simulink model "SPWM"  (R2016b)
settings: Solver=VariableStepAuto  StartTime=0.0  StopTime=0.1  RelTol=1e-3
libraries: powerlib x7, powerlib_meascontrol x2
settings Model: Creator=sususweet  LastModifiedBy=tangyq

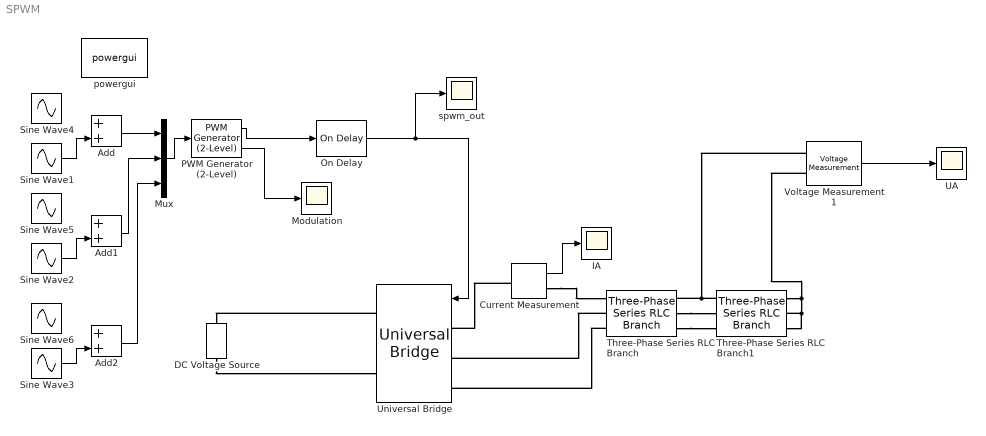
== system SPWM ==
  Add : Sum
  Add1 : Sum
  Add2 : Sum
  Current Measurement : powerlib/Measurements/Current Measurement  PhasorSimulation=off  OutputType=Complex  PSBequivalent=0
  DC Voltage Source : powerlib/Electrical Sources/DC Voltage Source  Amplitude=100  Measurements=Voltage
  IA : Scope
  Modulation : Scope
  Mux : Mux  Inputs=3
  On Delay : powerlib_meascontrol/Logic/On Delay  DelayType=On delay  delay=2e-6  ic=0  Ts=0
  PWM Generator (2-Level) : powerlib_meascontrol/Pulse & Signal Generators/PWM Generator (2-Level)  ModulatorType=Three-phase bridge (6 pulses)  ModulatorMode=Unsynchronized  Fc=10000  Pc=0  nF=27  MinMax="[ -1  1 ]"  SamplingTechnique=Symmetrical regular (single edge)  ModulatingSignals=off  m=1  Freq=50  Phase=0  Ts=0.00001  ShowCarrierOutport=on
  Sine Wave1 : Sin  Amplitude=0.8  Frequency=50*2*pi  SampleTime=0.00001
  Sine Wave2 : Sin  Amplitude=0.8  Frequency=50*2*pi  Phase=-2*pi/3  SampleTime=0.00001
  Sine Wave3 : Sin  Amplitude=0.8  Frequency=50*2*pi  Phase=2*pi/3  SampleTime=0.00001
  Sine Wave4 : Sin  Amplitude=0.8*0.1666  Frequency=150*2*pi  SampleTime=0.00001
  Sine Wave5 : Sin  Amplitude=0.8*0.1666  Frequency=150*2*pi  SampleTime=0.00001
  Sine Wave6 : Sin  Amplitude=0.8*0.1666  Frequency=150*2*pi  SampleTime=0.00001
  Three-Phase Series RLC Branch : powerlib/Elements/Three-Phase Series RLC Branch  LConnTagsString=A|B|C  RConnTagsString=A|B|C  BranchType=L  Resistance=20  Inductance=0.1  Capacitance=1e-6  Measurements=None
  Three-Phase Series RLC Branch1 : powerlib/Elements/Three-Phase Series RLC Branch  LConnTagsString=A|B|C  RConnTagsString=A|B|C  BranchType=R  Resistance=20  Inductance=0.05  Capacitance=1e-6  Measurements=None
  UA : Scope
  Universal Bridge : powerlib/Power Electronics/Universal Bridge  Arms=3  SnubberResistance=1e5  SnubberCapacitance=inf  Device=IGBT / Diodes  Ron=1e-3  Lon=0  ForwardVoltages="[  0  0  ]"  ForwardVoltage=0  GTOparameters=[ 10e-6 , 20e-6 ]  IGBTparameters=[ 1e-6 , 2e-6 ]  Measurements=None  Measurements_2=None  converterType=Rectifier
  Voltage Measurement1 : powerlib/Measurements/Voltage Measurement  PhasorSimulation=off  OutputType=Complex  PSBequivalent=0
  powergui : powerlib/powergui  Priority=1  SimulationMode=Continuous  SolverType=Tustin/Backward Euler (TBE)  SampleTime=50e-6  frequency=60  SPID=off  DisableSnubberDevices=off  DisableRonSwitches=off  DisableVfSwitches=off  SwTol=0  DisplayEquations=off  Interpol=off  ExternalGateDelay=off  methode=off  Ts=10  FunctionMessages=off  echomessages=off  HookPort=off  EnableUseOfTLC=off  x0status=blocks  frequencyindice=0  Pbase=100e6  ErrMax=1e-4  Iterations=50  UnitsV=kV  UnitsW=MW  buscounter=0  RestoreLinks=warning  ResistiveCurrentMeasurement=off  Frange=[0:2:500]  Ylog=off  Xlog=on  ShowGrid=off  save=off  variable=ZData  structure=UA  ZoomFFT=off  StartTime=0.02  cycles=2  DisplayStyle=2  fundamental=50  FreqAxis=off  MaxFrequency=5000  frequencyindicesteady=1  RmsSteady=1  display=off
  spwm_out : Scope
  wires:
  PWM Generator (2-Level)/1 -> On Delay/1
  Voltage Measurement1/1 -> UA/1
  On Delay/1 -> spwm_out/1, Universal Bridge/1
  Current Measurement/1 -> IA/1
  Add/1 -> Mux/1
  Sine Wave1/1 -> Add/2
  Add2/1 -> Mux/3
  Add1/1 -> Mux/2
  Sine Wave2/1 -> Add1/2
  Sine Wave3/1 -> Add2/2
  PWM Generator (2-Level)/2 -> Modulation/1
  Mux/1 -> PWM Generator (2-Level)/1
  connections:
  Universal Bridge/RConn1 -- DC Voltage Source/RConn1
  DC Voltage Source/LConn1 -- Universal Bridge/RConn2
  Three-Phase Series RLC Branch/LConn2 -- Universal Bridge/LConn2
  Current Measurement/LConn1 -- Universal Bridge/LConn1
  Three-Phase Series RLC Branch/LConn3 -- Universal Bridge/LConn3
  Current Measurement/RConn1 -- Three-Phase Series RLC Branch/LConn1
  Three-Phase Series RLC Branch1/RConn1 -- Voltage Measurement1/LConn2 -- Three-Phase Series RLC Branch1/RConn2 -- Three-Phase Series RLC Branch1/RConn3
  Three-Phase Series RLC Branch1/LConn1 -- Voltage Measurement1/LConn1 -- Three-Phase Series RLC Branch/RConn1
  Three-Phase Series RLC Branch/RConn2 -- Three-Phase Series RLC Branch1/LConn2
  Three-Phase Series RLC Branch/RConn3 -- Three-Phase Series RLC Branch1/LConn3
